simulink model "SAME70Q21B_MCPWM_MCLV2_PIM_DualShunt_R2018a"  (R2018a)
settings: Solver=FixedStepDiscrete  StartTime=0.0  StopTime=10.0  FixedStep=5e-5  RelTol=1e-3  EnableMultiTasking=on
undefined symbols (not defined in the file): A24, AD10, AD7, ADC0, DiscIntNeverNeededParam, gcbh, LQFP144, MCHP_AFEC_SAM7x_Callback, PA10, PA11, PA12, PA13, PA18, PA9, PB0, PB2, PB3, PD24, PD25, PD26, Pin, PWM0max0, SAME70Q21B, XData
libraries: MCHP_Blockset x10, simulink x9
(part 2 of 2)

== system SAME70Q21B_MCPWM_MCLV2_PIM_DualShunt_R2018a/Compute Voltage applied Within Alpha Beta Space1 ==
  Gain : Inport
  CosSin : Inport  Port=2
  DC Bus Voltage : Inport  Port=3
  Abs : Abs
  Delay : Delay  DelayLength=1  InitialCondition=0
  Product1 : Product  RndMeth=Zero  OutDataTypeStr=Inherit: Same as first input
  Product3 : Product  OutMin=[-24]  OutMax=[24]  RndMeth=Zero  OutDataTypeStr=Inherit: Same as first input
  ValphaBeta : Outport
  wires:
  Abs/1 -> Product1/2
  Gain/1 -> Abs/1
  CosSin/1 -> Delay/1
  Product3/1 -> ValphaBeta/1
  Product1/1 -> Product3/1
  DC Bus Voltage/1 -> Product3/2
  Delay/1 -> Product1/1

== system SAME70Q21B_MCPWM_MCLV2_PIM_DualShunt_R2018a/Invert Current Sign For reversed rotation1 ==
  Gain : Inport
  "Iab " : Inport  Port=2
  Compare To Zero1 : simulink/Logic and Bit Operations/Compare To Zero  relop=>=  OutDataTypeStr=boolean
  Gain4 : Gain  Gain=-1  RndMeth=Zero  SaturateOnIntegerOverflow=on  OutDataTypeStr=Inherit: Same as input
  Switch3 : Switch  Criteria=u2 ~= 0  Threshold=250
  "Iab_ " : Outport
  wires:
  "Iab "/1 -> Gain4/1, Switch3/1
  Gain/1 -> Compare To Zero1/1
  Switch3/1 -> "Iab_ "/1
  Compare To Zero1/1 -> Switch3/2
  Gain4/1 -> Switch3/3

== system SAME70Q21B_MCPWM_MCLV2_PIM_DualShunt_R2018a/OPEN Loop Startup sequence ==
  Constant1 : Constant  Value=149*2^-32  OutDataTypeStr=fixdt(0,32,32)  SampleTime=.00005
  Delay : Delay  DelayLength=1  InitialCondition=0
  Delay2 : Delay  DelayLength=1  InitialCondition=0
  Saturation : Saturate  UpperLimit=149*2^-32*3/.00005  LowerLimit=0
  Sum : Sum  Inputs=|++  AccumDataTypeStr=fixdt(0,32,32)  OutDataTypeStr=Inherit: Same as accumulator  RndMeth=Simplest
  Sum1 : Sum  Inputs=|++  AccumDataTypeStr=fixdt(0,32,32)  OutDataTypeStr=Inherit: Same as accumulator  RndMeth=Simplest
  Out1 : Outport
  wires:
  Delay/1 -> Sum/2
  Sum/1 -> Saturation/1  "Startup Ramp"
  Constant1/1 -> Sum/1
  Sum1/1 -> Out1/1, Delay2/1  "qAngle"
  Delay2/1 -> Sum1/2
  Saturation/1 -> Delay/1, Sum1/1

== system SAME70Q21B_MCPWM_MCLV2_PIM_DualShunt_R2018a/Scale ==
  In1 : Inport
  Data Type Conversion : DataTypeConversion  OutDataTypeStr=fixdt(1,32,31)
  Data Type Conversion1 : DataTypeConversion  OutDataTypeStr=fixdt(0,32,32)  ConvertRealWorld=Stored Integer (SI)
  Rate Transition2 : RateTransition
  Phase shift : Outport
  wires:
  In1/1 -> Data Type Conversion/1
  Data Type Conversion/1 -> Data Type Conversion1/1
  Data Type Conversion1/1 -> Rate Transition2/1
  Rate Transition2/1 -> Phase shift/1

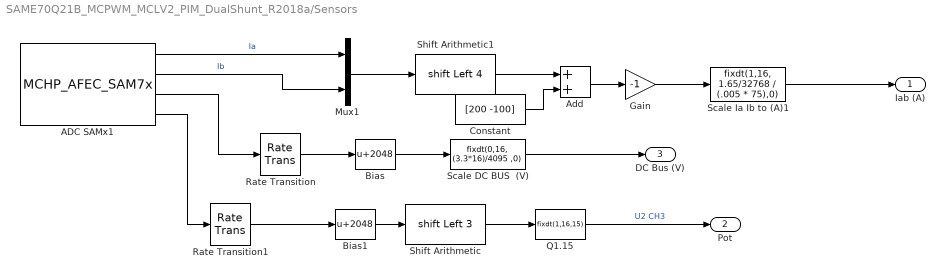
== system SAME70Q21B_MCPWM_MCLV2_PIM_DualShunt_R2018a/Sensors ==
  ADC SAMx1 : S-Function  Priority=-2000  AncestorBlock=MCHP_Blockset/Analog IO/ADC SAMx7  LoadFcn=|  InitFcn=MCHP_AFEC_SAM7x_Callback(gcbh,'InitFcn');  FunctionName=MCHP_AFEC_SAM7x  Parameters=MCHP_AFEC_SAM7x_Callback(gcbh,'S_INPUT'),MCHP_AFEC_SAM7x_Callback(gcbh,'S_OUTPUT'),MCHP_AFEC_SAM7x_Callback(gcbh,'S_INPUT_Size'),MCHP_AFEC_SAM7x_Callback(gcbh,'S_OUTPUT_Size'),MCHP_AFEC_SAM7x_Callback(gcbh,'S_ListCustomDatatype'),SampleTime,0  SFunctionDeploymentMode=off  EnableBusSupport=off  mask(ADC for SAMx7){AFECx=AFE Controller 0, SIGNMODE_SingleEnded=Signed    (int16), SIGNMODE_Differential=Unsigned (uint16), AFEC0_seq0=Dynamic Options, AFEC0_seq0_TXT=AD0 / PD30   &   AD6 / PA17, AFEC1_seq0=Dynamic Options, AFEC1_seq0_TXT=Not used, AFEC0_seq1=Dynamic Options, AFEC0_seq1_TXT=AD7 / PA18, AFEC1_seq1=Dynamic Options, AFEC1_seq1_TXT=Not used, AFEC0_seq2=Dynamic Options, AFEC0_seq2_TXT=AD10 / PB0, AFEC1_seq2=Dynamic Options, AFEC1_seq2_TXT=Not used, AFEC0_seq3=Dynamic Options, AFEC0_seq3_TXT=Not used, AFEC1_seq3=Dynamic Options, AFEC1_seq3_TXT=Not used, AFEC0_seq4=Dynamic Options, AFEC0_seq4_TXT=Not used, AFEC1_seq4=Dynamic Options, AFEC1_seq4_TXT=Not used, AFEC0_seq5=Dynamic Options, AFEC0_seq5_TXT=Not used, AFEC1_seq5=Dynamic Options, AFEC1_seq5_TXT=Not used, AFEC0_seq6=Dynamic Options, AFEC0_seq6_TXT=Not used, AFEC1_seq6=Dynamic Options, AFEC1_seq6_TXT=Not used, AFEC0_seq7=Dynamic Options, AFEC0_seq7_TXT=Not used, AFEC1_seq7=Dynamic Options, AFEC1_seq7_TXT=Not used, AFEC0_seq8=Dynamic Options, AFEC0_seq8_TXT=Not used, AFEC1_seq8=Dynamic Options, AFEC1_seq8_TXT=Not used, AFEC0_seq9=Dynamic Options, AFEC0_seq9_TXT=Not used, AFEC1_seq9=Dynamic Options, AFEC1_seq9_TXT=Not used, AFEC0_seq10=Dynamic Options, AFEC0_seq10_TXT=Not used, AFEC1_seq10=Dynamic Options, AFEC1_seq10_TXT=Not used, AFEC0_seq11=Dynamic Options, AFEC0_seq11_TXT=Not used, AFEC1_seq11=Dynamic Options, AFEC1_seq11_TXT=Not used, SampleTime=.00005, S_INPUT=[-1], S_INPUT_Size=[3], S_OUTPUT=[], S_OUTPUT_Size=[], S_ListCustomDatatype=S.S_ListCustomDatatype={};, evalin_ws=, MCHP_AFECC_CLOCK_REQUEST='', MCHP_AFECC_CLOCK_RESULT='', MCHP_USER_INTERRUPTS=0, MCHP_PORT={AD0 AFEC0}{AD0}15:2:P126;{AD6 AFEC0}{AD6}15:2:P17;{AD7 AFEC0}{AD7}15:2:P18;{AD10 AFEC0}{AD10}15:2:P32;, MCHP_MASTERLINK=SAME70Q21B_MCPWM_MCLV2_PIM_DualShunt_R2018a/Microchip Master, Rin=< 200 Ohm, RES=12-bit Standard, AFEC0_Synchronisation=Triggered by user defined source, AFEC0_Trig=PWM0 event line 0, AFEC0_TrigTimeStep=on, AFEC1_Synchronisation=Triggered by user defined source, AFEC1_Trig=PWM1 event line 0, AFEC1_TrigTimeStep=off, ADC_TrigInfo=0, AFEC0_seq0_GAIN=1, AFEC1_seq0_GAIN=1, AFEC0_seq1_GAIN=1, AFEC1_seq1_GAIN=1, AFEC0_seq2_GAIN=1, AFEC1_seq2_GAIN=1, AFEC0_seq3_GAIN=1, AFEC1_seq3_GAIN=1, AFEC0_seq4_GAIN=1, AFEC1_seq4_GAIN=1, AFEC0_seq5_GAIN=1, AFEC1_seq5_GAIN=1, AFEC0_seq6_GAIN=1, AFEC1_seq6_GAIN=1, AFEC0_seq7_GAIN=1, AFEC1_seq7_GAIN=1, AFEC0_seq8_GAIN=1, AFEC1_seq8_GAIN=1, AFEC0_seq9_GAIN=1, AFEC1_seq9_GAIN=1, AFEC0_seq10_GAIN=1, AFEC1_seq10_GAIN=1, AFEC0_seq11_GAIN=1, AFEC1_seq11_GAIN=1, AFEC0_seq0_OFFSET=0, AFEC1_seq0_OFFSET=0, AFEC0_seq1_OFFSET=0, AFEC1_seq1_OFFSET=0, AFEC0_seq2_OFFSET=0, AFEC1_seq2_OFFSET=0, AFEC0_seq3_OFFSET=0, AFEC1_seq3_OFFSET=0, AFEC0_seq4_OFFSET=0, AFEC1_seq4_OFFSET=0, AFEC0_seq5_OFFSET=0, AFEC1_seq5_OFFSET=0, AFEC0_seq6_OFFSET=0, AFEC1_seq6_OFFSET=0, AFEC0_seq7_OFFSET=0, AFEC1_seq7_OFFSET=0, AFEC0_seq8_OFFSET=0, AFEC1_seq8_OFFSET=0, AFEC0_seq9_OFFSET=0, AFEC1_seq9_OFFSET=0, AFEC0_seq10_OFFSET=0, AFEC1_seq10_OFFSET=0, AFEC0_seq11_OFFSET=0, AFEC1_seq11_OFFSET=0}
      | txt = get_param(gcbh,'evalin_ws');
      | evalin('base',txt);
      mask prompts: AFECx "Select ADC (AFEC) Controller :"; SIGNMODE_SingleEnded "Single-Ended conversion output are"; SIGNMODE_Differential "Differential conversions output are"; AFEC0_seq0 "AFEC0 seq 0"; AFEC0_seq0_TXT "sequence x"; AFEC1_seq0 "AFEC1 seq 0"; AFEC1_seq0_TXT "sequence x"; AFEC0_seq1 "AFEC0 seq 1"; AFEC0_seq1_TXT "sequence x"; AFEC1_seq1 "AFEC1 seq 1"; AFEC1_seq1_TXT "sequence x"; AFEC0_seq2 "AFEC0 seq 2"; AFEC0_seq2_TXT "sequence x"; AFEC1_seq2 "AFEC1 seq 2"; AFEC1_seq2_TXT "sequence x"; AFEC0_seq3 "AFEC0 seq 3"; AFEC0_seq3_TXT "sequence x"; AFEC1_seq3 "AFEC1 seq 3"; AFEC1_seq3_TXT "sequence x"; AFEC0_seq4 "AFEC0 seq 4"; AFEC0_seq4_TXT "sequence x"; AFEC1_seq4 "AFEC1 seq 4"; AFEC1_seq4_TXT "sequence x"; AFEC0_seq5 "AFEC0 seq 5"; AFEC0_seq5_TXT "sequence x"; AFEC1_seq5 "AFEC1 seq 5"; AFEC1_seq5_TXT "sequence x"; AFEC0_seq6 "AFEC0 seq 6"; AFEC0_seq6_TXT "sequence x"; AFEC1_seq6 "AFEC1 seq 6"; AFEC1_seq6_TXT "sequence x"; AFEC0_seq7 "AFEC0 seq 7"; AFEC0_seq7_TXT "sequence x"; AFEC1_seq7 "AFEC1 seq 7"; AFEC1_seq7_TXT "sequence x"; AFEC0_seq8 "AFEC0 seq 8"; AFEC0_seq8_TXT "sequence x"; AFEC1_seq8 "AFEC1 seq 8"; AFEC1_seq8_TXT "sequence x"; AFEC0_seq9 "AFEC0 seq 9"; AFEC0_seq9_TXT "sequence x"; AFEC1_seq9 "AFEC1 seq 9"; AFEC1_seq9_TXT "sequence x"; AFEC0_seq10 "AFEC0 seq 10"; AFEC0_seq10_TXT "sequence x"; AFEC1_seq10 "AFEC1 seq 10"; AFEC1_seq10_TXT "sequence x"; AFEC0_seq11 "AFEC0 seq 11"; AFEC0_seq11_TXT "sequence x"; AFEC1_seq11 "AFEC1 seq 11"; AFEC1_seq11_TXT "sequence x"; SampleTime "Block output sample time"; Rin "Input impedance (Tsamp=400(ns) ; Tconv=213.33(ns))"; RES "Resolution and Digital Filter"; AFEC0_Synchronisation "ADC Sample and Conversion"; AFEC0_Trig "User defined trigger (AFEC0):"; AFEC0_TrigTimeStep "The model base Time Step is triggered by the the last ADC conversion using this trigger"; AFEC1_Synchronisation "ADC Sample and Conversion"; AFEC1_Trig "User defined trigger (AFEC1):"; AFEC1_TrigTimeStep "The model base Time Step is triggered by the the last ADC conversion using this trigger"; ADC_TrigInfo "ADC Trigger Info"; AFEC0_seq0_GAIN "AD0 - PD30 Gain"; AFEC1_seq0_GAIN "AD0 - PB1 Gain"; AFEC0_seq1_GAIN "AD1 - PA21 Gain"; AFEC1_seq1_GAIN "AD1 - PC13 Gain"; AFEC0_seq2_GAIN "AD2 - PB3 Gain"; AFEC1_seq2_GAIN "AD2 - PC15 Gain"; AFEC0_seq3_GAIN "AD3 - PE5 Gain"; AFEC1_seq3_GAIN "AD3 - PC12 Gain"; AFEC0_seq4_GAIN "AD4 - PE4 Gain"; AFEC1_seq4_GAIN "AD4 - PC29 Gain"; AFEC0_seq5_GAIN "AD5 - PB2 Gain"; AFEC1_seq5_GAIN "AD5 - PC30 Gain"; AFEC0_seq6_GAIN "AD6 - PA17 Gain"; AFEC1_seq6_GAIN "AD6 - PC31 Gain"; AFEC0_seq7_GAIN "AD7 - PA18 Gain"; AFEC1_seq7_GAIN "AD7 - PC26 Gain"; AFEC0_seq8_GAIN "AD8 - PA19 Gain"; AFEC1_seq8_GAIN "AD8 - PC27 Gain"; AFEC0_seq9_GAIN "AD9 - PA20 Gain"; AFEC1_seq9_GAIN "AD9 - PC0 Gain"; AFEC0_seq10_GAIN "AD10 - PB0 Gain"; AFEC1_seq10_GAIN "AD10 - PE3 Gain"; AFEC0_seq11_GAIN "AD11 - T Gain"; AFEC1_seq11_GAIN "AD11 - PE0 Gain"; AFEC0_seq0_OFFSET "AD0 - PD30 Offset within [-512 511]"; AFEC1_seq0_OFFSET "AD0 - PB1 Offset within [-512 511]"; AFEC0_seq1_OFFSET "AD1 - PA21 Offset within [-512 511]"; AFEC1_seq1_OFFSET "AD1 - PC13 Offset within [-512 511]"; AFEC0_seq2_OFFSET "AD2 - PB3 Offset within [-512 511]"; AFEC1_seq2_OFFSET "AD2 - PC15 Offset within [-512 511]"; AFEC0_seq3_OFFSET "AD3 - PE5 Offset within [-512 511]"; AFEC1_seq3_OFFSET "AD3 - PC12 Offset within [-512 511]"; AFEC0_seq4_OFFSET "AD4 - PE4 Offset within [-512 511]"; AFEC1_seq4_OFFSET "AD4 - PC29 Offset within [-512 511]"; AFEC0_seq5_OFFSET "AD5 - PB2 Offset within [-512 511]"; AFEC1_seq5_OFFSET "AD5 - PC30 Offset within [-512 511]"; AFEC0_seq6_OFFSET "AD6 - PA17 Offset within [-512 511]"; AFEC1_seq6_OFFSET "AD6 - PC31 Offset within [-512 511]"; AFEC0_seq7_OFFSET "AD7 - PA18 Offset within [-512 511]"; AFEC1_seq7_OFFSET "AD7 - PC26 Offset within [-512 511]"; AFEC0_seq8_OFFSET "AD8 - PA19 Offset within [-512 511]"; AFEC1_seq8_OFFSET "AD8 - PC27 Offset within [-512 511]"; AFEC0_seq9_OFFSET "AD9 - PA20 Offset within [-512 511]"; AFEC1_seq9_OFFSET "AD9 - PC0 Offset within [-512 511]"; AFEC0_seq10_OFFSET "AD10 - PB0 Offset within [-512 511]"; AFEC1_seq10_OFFSET "AD10 - PE3 Offset within [-512 511]"; AFEC0_seq11_OFFSET "AD11 - T Offset within [-512 511]"; AFEC1_seq11_OFFSET "AD11 - PE0 Offset within [-512 511]"
      mask help:
      | Configure the Analog Front End Controller (AFEC).
      |
      | Two AFEC modules can be configured independantly using two ADC blocks.
      | They will have common parameters when set with one common block.
      |
      | The 11 analog input pins are different for each AFEC.
      |
      | The sequence set in the block is listed in sampling chronological order.
      mask init:
      | MCHP_AFEC_SAM7x_Callback(gcbh,'INITIALISATION');
      settings: CopyFcn=MCHP_AFEC_SAM7x_Callback(gcbh,'CopyFcn');  PreSaveFcn=MCHP_Fun.PreSaveFcn_DynamicOptions(gcbh);  OpenFcn=MCHP_AFEC_SAM7x_Callback(gcbh,'OPEN');
      mask TypeOptions AFECx: AFE Controller 0 | AFE Controller 1 | AFE Controller 0 & 1
      mask Callback AFECx: MCHP_AFEC_SAM7x_Callback(gcbh,'UpdateGUI');
      mask TypeOptions SIGNMODE_SingleEnded: Unsigned (uint16) | Signed    (int16)
      mask TypeOptions SIGNMODE_Differential: Unsigned (uint16) | Signed    (int16)
      mask TypeOptions AFEC0_seq0: Dynamic Options
      mask Callback AFEC0_seq0: MCHP_AFEC_SAM7x_Callback(gcbh,'UpdateGUI');
      mask Callback AFEC0_seq0_TXT: MCHP_AFEC_SAM7x_Callback(gcbh,'UpdateGUI');
      mask TypeOptions AFEC1_seq0: Dynamic Options
      mask Callback AFEC1_seq0: MCHP_AFEC_SAM7x_Callback(gcbh,'UpdateGUI');
      mask Callback AFEC1_seq0_TXT: MCHP_AFEC_SAM7x_Callback(gcbh,'UpdateGUI');
      mask TypeOptions AFEC0_seq1: Dynamic Options
      mask Callback AFEC0_seq1: MCHP_AFEC_SAM7x_Callback(gcbh,'UpdateGUI');
      mask Callback AFEC0_seq1_TXT: MCHP_AFEC_SAM7x_Callback(gcbh,'UpdateGUI');
      mask TypeOptions AFEC1_seq1: Dynamic Options
      mask Callback AFEC1_seq1: MCHP_AFEC_SAM7x_Callback(gcbh,'UpdateGUI');
      mask Callback AFEC1_seq1_TXT: MCHP_AFEC_SAM7x_Callback(gcbh,'UpdateGUI');
      mask TypeOptions AFEC0_seq2: Dynamic Options
      mask Callback AFEC0_seq2_TXT: MCHP_AFEC_SAM7x_Callback(gcbh,'UpdateGUI');
      mask TypeOptions AFEC1_seq2: Dynamic Options
      mask Callback AFEC1_seq2_TXT: MCHP_AFEC_SAM7x_Callback(gcbh,'UpdateGUI');
      mask TypeOptions AFEC0_seq3: Dynamic Options
      mask Callback AFEC0_seq3: MCHP_AFEC_SAM7x_Callback(gcbh,'UpdateGUI');
      mask Callback AFEC0_seq3_TXT: MCHP_AFEC_SAM7x_Callback(gcbh,'UpdateGUI');
      mask TypeOptions AFEC1_seq3: Dynamic Options
      mask Callback AFEC1_seq3: MCHP_AFEC_SAM7x_Callback(gcbh,'UpdateGUI');
      mask Callback AFEC1_seq3_TXT: MCHP_AFEC_SAM7x_Callback(gcbh,'UpdateGUI');
      mask TypeOptions AFEC0_seq4: Dynamic Options
      mask Callback AFEC0_seq4: MCHP_AFEC_SAM7x_Callback(gcbh,'UpdateGUI');
      mask Callback AFEC0_seq4_TXT: MCHP_AFEC_SAM7x_Callback(gcbh,'UpdateGUI');
      mask TypeOptions AFEC1_seq4: Dynamic Options
      mask Callback AFEC1_seq4: MCHP_AFEC_SAM7x_Callback(gcbh,'UpdateGUI');
      mask Callback AFEC1_seq4_TXT: MCHP_AFEC_SAM7x_Callback(gcbh,'UpdateGUI');
      mask TypeOptions AFEC0_seq5: Dynamic Options
      mask Callback AFEC0_seq5: MCHP_AFEC_SAM7x_Callback(gcbh,'UpdateGUI');
      mask Callback AFEC0_seq5_TXT: MCHP_AFEC_SAM7x_Callback(gcbh,'UpdateGUI');
      mask TypeOptions AFEC1_seq5: Dynamic Options
      mask Callback AFEC1_seq5: MCHP_AFEC_SAM7x_Callback(gcbh,'UpdateGUI');
      mask Callback AFEC1_seq5_TXT: MCHP_AFEC_SAM7x_Callback(gcbh,'UpdateGUI');
      mask TypeOptions AFEC0_seq6: Dynamic Options
      mask Callback AFEC0_seq6: MCHP_AFEC_SAM7x_Callback(gcbh,'UpdateGUI');
      mask Callback AFEC0_seq6_TXT: MCHP_AFEC_SAM7x_Callback(gcbh,'UpdateGUI');
      mask TypeOptions AFEC1_seq6: Dynamic Options
      mask Callback AFEC1_seq6: MCHP_AFEC_SAM7x_Callback(gcbh,'UpdateGUI');
      mask Callback AFEC1_seq6_TXT: MCHP_AFEC_SAM7x_Callback(gcbh,'UpdateGUI');
      mask TypeOptions AFEC0_seq7: Dynamic Options
      mask Callback AFEC0_seq7: MCHP_AFEC_SAM7x_Callback(gcbh,'UpdateGUI');
      mask Callback AFEC0_seq7_TXT: MCHP_AFEC_SAM7x_Callback(gcbh,'UpdateGUI');
      mask TypeOptions AFEC1_seq7: Dynamic Options
      mask Callback AFEC1_seq7: MCHP_AFEC_SAM7x_Callback(gcbh,'UpdateGUI');
      mask Callback AFEC1_seq7_TXT: MCHP_AFEC_SAM7x_Callback(gcbh,'UpdateGUI');
      mask TypeOptions AFEC0_seq8: Dynamic Options
      mask Callback AFEC0_seq8: MCHP_AFEC_SAM7x_Callback(gcbh,'UpdateGUI');
      mask Callback AFEC0_seq8_TXT: MCHP_AFEC_SAM7x_Callback(gcbh,'UpdateGUI');
      mask TypeOptions AFEC1_seq8: Dynamic Options
      mask Callback AFEC1_seq8: MCHP_AFEC_SAM7x_Callback(gcbh,'UpdateGUI');
      mask Callback AFEC1_seq8_TXT: MCHP_AFEC_SAM7x_Callback(gcbh,'UpdateGUI');
      mask TypeOptions AFEC0_seq9: Dynamic Options
      mask Callback AFEC0_seq9: MCHP_AFEC_SAM7x_Callback(gcbh,'UpdateGUI');
      mask Callback AFEC0_seq9_TXT: MCHP_AFEC_SAM7x_Callback(gcbh,'UpdateGUI');
      mask TypeOptions AFEC1_seq9: Dynamic Options
      mask Callback AFEC1_seq9: MCHP_AFEC_SAM7x_Callback(gcbh,'UpdateGUI');
      mask Callback AFEC1_seq9_TXT: MCHP_AFEC_SAM7x_Callback(gcbh,'UpdateGUI');
      mask TypeOptions AFEC0_seq10: Dynamic Options
      mask Callback AFEC0_seq10: MCHP_AFEC_SAM7x_Callback(gcbh,'UpdateGUI');
      mask Callback AFEC0_seq10_TXT: MCHP_AFEC_SAM7x_Callback(gcbh,'UpdateGUI');
      mask TypeOptions AFEC1_seq10: Dynamic Options
      mask Callback AFEC1_seq10: MCHP_AFEC_SAM7x_Callback(gcbh,'UpdateGUI');
      mask Callback AFEC1_seq10_TXT: MCHP_AFEC_SAM7x_Callback(gcbh,'UpdateGUI');
      mask TypeOptions AFEC0_seq11: Dynamic Options
      mask Callback AFEC0_seq11: MCHP_AFEC_SAM7x_Callback(gcbh,'UpdateGUI');
      mask Callback AFEC0_seq11_TXT: MCHP_AFEC_SAM7x_Callback(gcbh,'UpdateGUI');
      mask TypeOptions AFEC1_seq11: Dynamic Options
      mask Callback AFEC1_seq11: MCHP_AFEC_SAM7x_Callback(gcbh,'UpdateGUI');
      mask Callback AFEC1_seq11_TXT: MCHP_AFEC_SAM7x_Callback(gcbh,'UpdateGUI');
      mask TypeOptions Rin: < 200 Ohm | < 500 Ohm | < 1    kOhm | < 2    kOhm | < 5    kOhm | < 10   kOhm | < 20   kOhm | < 50   kOhm | < 100  kOhm | < 200  kOhm | < 500  kOhm | max sampling time
      mask TypeOptions RES: 10-bit Low Resolution | 12-bit Standard | 13-bit (Average 4 conversions) | 14-bit (Average 16 conversions) | 15-bit (Average 64 conversions) | 16-bit (Average 256 conversions)
      mask TypeOptions AFEC0_Synchronisation: Software triggered after reading last converted value | Triggered by user defined source | Free Run. Output is last converted value
      mask Callback AFEC0_Synchronisation: MCHP_AFEC_SAM7x_Callback(gcbh,'UpdateGUI');
      mask TypeOptions AFEC0_Trig: AFE0_ADTRG input pin | PWM0 event line 0 | PWM0 event line 1 | Timer Counter Channel 0 | Timer Counter Channel 1 | Timer Counter Channel 2 | Analog Comparator
      mask TypeOptions AFEC1_Synchronisation: Software triggered after reading last converted value | Triggered by user defined source | Free Run. Output is last converted value
      mask Callback AFEC1_Synchronisation: MCHP_AFEC_SAM7x_Callback(gcbh,'UpdateGUI');
      mask TypeOptions AFEC1_Trig: AFE1_ADTRG input pin | PWM1 event line 0 | PWM1 event line 1 | Timer Counter Channel 3 | Timer Counter Channel 4 | Timer Counter Channel 5 | Analog Comparator
      mask TypeOptions AFEC0_seq0_GAIN: 1 | 2 | 4
      mask TypeOptions AFEC1_seq0_GAIN: 1 | 2 | 4
      mask TypeOptions AFEC0_seq1_GAIN: 1 | 2 | 4
      mask TypeOptions AFEC1_seq1_GAIN: 1 | 2 | 4
      mask TypeOptions AFEC0_seq2_GAIN: 1 | 2 | 4
      mask TypeOptions AFEC1_seq2_GAIN: 1 | 2 | 4
      mask TypeOptions AFEC0_seq3_GAIN: 1 | 2 | 4
      mask TypeOptions AFEC1_seq3_GAIN: 1 | 2 | 4
      mask TypeOptions AFEC0_seq4_GAIN: 1 | 2 | 4
      mask TypeOptions AFEC1_seq4_GAIN: 1 | 2 | 4
      mask TypeOptions AFEC0_seq5_GAIN: 1 | 2 | 4
      mask TypeOptions AFEC1_seq5_GAIN: 1 | 2 | 4
      mask TypeOptions AFEC0_seq6_GAIN: 1 | 2 | 4
      mask TypeOptions AFEC1_seq6_GAIN: 1 | 2 | 4
      mask TypeOptions AFEC0_seq7_GAIN: 1 | 2 | 4
      mask TypeOptions AFEC1_seq7_GAIN: 1 | 2 | 4
      mask TypeOptions AFEC0_seq8_GAIN: 1 | 2 | 4
      mask TypeOptions AFEC1_seq8_GAIN: 1 | 2 | 4
      mask TypeOptions AFEC0_seq9_GAIN: 1 | 2 | 4
      mask TypeOptions AFEC1_seq9_GAIN: 1 | 2 | 4
      mask TypeOptions AFEC0_seq10_GAIN: 1 | 2 | 4
      mask TypeOptions AFEC1_seq10_GAIN: 1 | 2 | 4
      mask TypeOptions AFEC0_seq11_GAIN: 1 | 2 | 4
      mask TypeOptions AFEC1_seq11_GAIN: 1 | 2 | 4
      mask DialogControl ParameterTabVar0 Prompt: Analog Channels
      mask DialogControl ParameterTabVar01 Prompt: Options
      mask DialogControl ParameterTabVar012 Prompt: Gain
      mask DialogControl ParameterTabVar0123 Prompt: Offset
      mask Display:
      | fprintf(['AFEC SAMx7\n' AFECx(4:end)]);
      | port_label('output',1,'PD30');
      | port_label('output',2,'PA17');
      | port_label('output',3,'PA18');
      | port_label('output',4,'PB0');
  Add : Sum  SaturateOnIntegerOverflow=on  OutDataTypeStr=Inherit: Same as first input
  Bias : Bias  Bias=2048
  Bias1 : Bias  Bias=2048
  Constant : Constant  Value=[200 -100]  OutDataTypeStr=int16
  Gain : Gain  Gain=-1  SaturateOnIntegerOverflow=on  OutDataTypeStr=Inherit: Same as input
  Mux1 : Mux  Inputs=2
  Q1.15 : DataTypeConversion  OutDataTypeStr=fixdt(1,16,15)  ConvertRealWorld=Stored Integer (SI)
  Rate Transition : RateTransition  OutPortSampleTime=.001
  Rate Transition1 : RateTransition  OutPortSampleTime=.001
  Scale DC BUS  (V) : DataTypeConversion  OutDataTypeStr=fixdt(0,16, (3.3*16)/4095 ,0)  ConvertRealWorld=Stored Integer (SI)
  Scale Ia Ib to (A)1 : DataTypeConversion  OutDataTypeStr=fixdt(1,16, 1.65/32768 / (.005 * 75),0)  ConvertRealWorld=Stored Integer (SI)
  Shift Arithmetic : ArithShift  BitShiftNumber=3  BitShiftDirection=Left
  Shift Arithmetic1 : ArithShift  BitShiftNumber=4  BitShiftDirection=Left
  Iab (A) : Outport
  Pot : Outport  Port=2
  DC Bus (V) : Outport  Port=3
  wires:
  Q1.15/1 -> Pot/1  "U2 CH3"
  Mux1/1 -> Shift Arithmetic1/1
  Scale Ia Ib to (A)1/1 -> Iab (A)/1
  Scale DC BUS  (V)/1 -> DC Bus (V)/1
  ADC SAMx1/4 -> Rate Transition1/1
  Shift Arithmetic/1 -> Q1.15/1
  Bias/1 -> Scale DC BUS  (V)/1
  ADC SAMx1/3 -> Rate Transition/1
  Bias1/1 -> Shift Arithmetic/1
  Rate Transition/1 -> Bias/1
  Rate Transition1/1 -> Bias1/1
  ADC SAMx1/2 -> Mux1/2  "Ib"
  Shift Arithmetic1/1 -> Add/1
  Add/1 -> Gain/1
  ADC SAMx1/1 -> Mux1/1  "Ia"
  Constant/1 -> Add/2
  Gain/1 -> Scale Ia Ib to (A)1/1

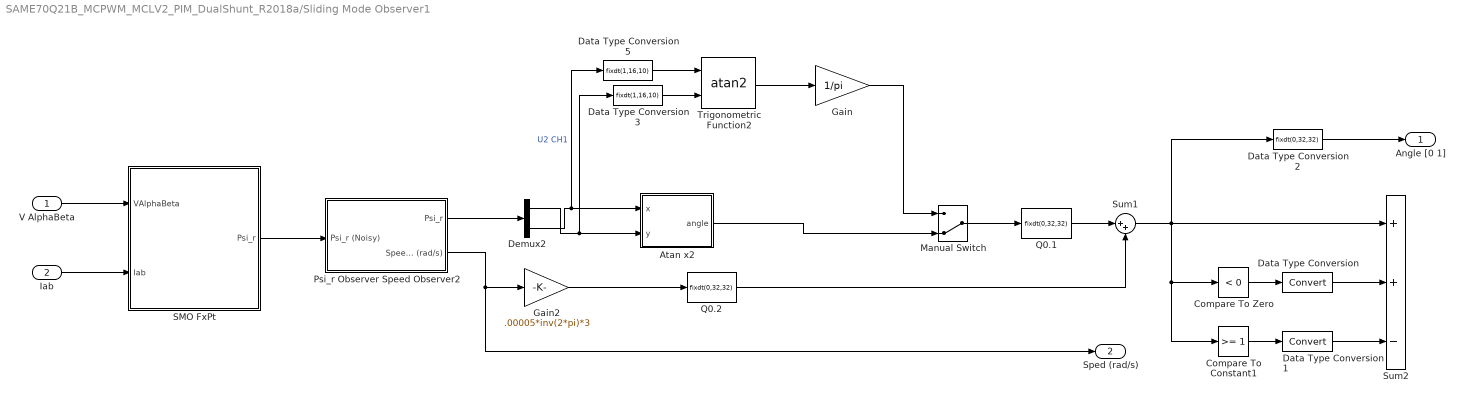
== system SAME70Q21B_MCPWM_MCLV2_PIM_DualShunt_R2018a/Sliding Mode Observer1 ==
  V AlphaBeta : Inport
  Iab : Inport  Port=2
  Atan x2 : Subsystem  AncestorBlock=Lib_MCHP_BLKDEMO_Motor/Atan x2
  Compare To Constant1 : simulink/Logic and Bit Operations/Compare To Constant  relop=>=  const=1  OutDataTypeStr=boolean
  Compare To Zero : simulink/Logic and Bit Operations/Compare To Zero  relop=<  OutDataTypeStr=boolean
  Data Type Conversion : DataTypeConversion  RndMeth=Zero
  Data Type Conversion1 : DataTypeConversion  RndMeth=Zero
  Data Type Conversion2 : DataTypeConversion  OutDataTypeStr=fixdt(0,32,32)  RndMeth=Zero
  Data Type Conversion3 : DataTypeConversion  OutDataTypeStr=fixdt(1,16,10)  RndMeth=Zero
  Data Type Conversion5 : DataTypeConversion  OutDataTypeStr=fixdt(1,16,10)  RndMeth=Zero
  Demux2 : Demux  Outputs=2
  Gain : Gain  Gain=1/pi  OutDataTypeStr=fixdt(1,32,31)  RndMeth=Zero
  Gain2 : Gain  Gain=.00005*inv(2*pi)*3  OutDataTypeStr=fixdt(1,32,31)  RndMeth=Zero
  Manual Switch : ManualSwitch  CurrentSetting=0
  Psi_r Observer Speed Observer2 : Subsystem
  Q0.1 : DataTypeConversion  OutDataTypeStr=fixdt(0,32,32)  ConvertRealWorld=Stored Integer (SI)  RndMeth=Simplest
  Q0.2 : DataTypeConversion  OutDataTypeStr=fixdt(0,32,32)  ConvertRealWorld=Stored Integer (SI)  RndMeth=Simplest
  SMO FxPt : Subsystem
  Sum1 : Sum  Inputs=|++  OutDataTypeStr=Inherit: Same as accumulator  RndMeth=Zero
  Sum2 : Sum  Inputs=++-  OutDataTypeStr=Inherit: Same as accumulator  RndMeth=Zero
  Trigonometric Function2 : Trigonometry  Operator=atan2  ApproximationMethod=CORDIC  NumberOfIterations=10  OutputSignalType=real
  Angle [0 1] : Outport
  Sped (rad/s) : Outport  Port=2
  wires:
  Data Type Conversion2/1 -> Angle [0 1]/1
  Trigonometric Function2/1 -> Gain/1
  Data Type Conversion1/1 -> Sum2/3
  Data Type Conversion/1 -> Sum2/2
  Compare To Constant1/1 -> Data Type Conversion1/1
  Compare To Zero/1 -> Data Type Conversion/1
  Gain/1 -> Manual Switch/1
  Atan x2/1(angle) -> Manual Switch/2
  Demux2/2 -> Data Type Conversion5/1, Atan x2/1(x)  "U2 CH1"
  Manual Switch/1 -> Q0.1/1
  Sum1/1 -> Compare To Zero/1, Compare To Constant1/1, Data Type Conversion2/1, Sum2/1
  Iab/1 -> SMO FxPt/2(Iab)
  Psi_r Observer Speed Observer2/2(Speed we (rad/s)) -> Gain2/1, Sped (rad/s)/1
  SMO FxPt/1(Psi_r) -> Psi_r Observer Speed Observer2/1(Psi_r (Noisy))
  V AlphaBeta/1 -> SMO FxPt/1(VAlphaBeta)
  Psi_r Observer Speed Observer2/1(Psi_r) -> Demux2/1
  Demux2/1 -> Atan x2/2(y), Data Type Conversion3/1
  Gain2/1 -> Q0.2/1
  Q0.1/1 -> Sum1/1
  Data Type Conversion5/1 -> Trigonometric Function2/1
  Data Type Conversion3/1 -> Trigonometric Function2/2
  Q0.2/1 -> Sum1/2

== system SAME70Q21B_MCPWM_MCLV2_PIM_DualShunt_R2018a/Subsystem1 ==
  OL : Inport
  CL : Inport  Port=2
  Rate Transition10 : RateTransition
  Switch Startup ramp Angle then Estimated Angle or QEI : Switch  Criteria=u2 ~= 0  Threshold=250
  OL/CL : Outport
  wires:
  [CL] -> Rate Transition10/1
  Rate Transition10/1 -> Switch Startup ramp Angle then Estimated Angle or QEI/2
  Switch Startup ramp Angle then Estimated Angle or QEI/1 -> OL/CL/1
  OL/1 -> Switch Startup ramp Angle then Estimated Angle or QEI/3
  CL/1 -> Switch Startup ramp Angle then Estimated Angle or QEI/1

== system SAME70Q21B_MCPWM_MCLV2_PIM_DualShunt_R2018a/Subsystem2 ==
  CL : Inport
  OL : Inport  Port=2
  Rate Transition10 : RateTransition
  Switch Startup ramp Angle then Estimated Angle or QEI : Switch  Criteria=u2 ~= 0  Threshold=250
  OL/CL : Outport
  wires:
  CL/1 -> Switch Startup ramp Angle then Estimated Angle or QEI/1
  OL/1 -> Switch Startup ramp Angle then Estimated Angle or QEI/3
  Rate Transition10/1 -> Switch Startup ramp Angle then Estimated Angle or QEI/2
  [CL] -> Rate Transition10/1
  Switch Startup ramp Angle then Estimated Angle or QEI/1 -> OL/CL/1

== system SAME70Q21B_MCPWM_MCLV2_PIM_DualShunt_R2018a/Switch from OpenLoop to Closed Loop ==
  Speed : Inport
  Abs : Abs
  Delay1 : Delay  DelayLength=1  InitialCondition=[0]
  Logical Operator1 : Logic  Operator=OR  AllPortsSameDT=off  OutDataTypeStr=boolean
  Rate Transition8 : RateTransition  OutPortSampleTime=.01
  Switching Speed (rad/s Electrical) : simulink/Logic and Bit Operations/Compare To Constant  relop=>  const=100  OutDataTypeStr=boolean
  ClosedLoop 0/1 : Outport
  wires:
  Abs/1 -> Switching Speed (rad/s Electrical)/1
  Speed/1 -> Rate Transition8/1
  Rate Transition8/1 -> Abs/1
  Delay1/1 -> Logical Operator1/1, ClosedLoop 0/1/1
  Switching Speed (rad/s Electrical)/1 -> Logical Operator1/2
  Logical Operator1/1 -> Delay1/1

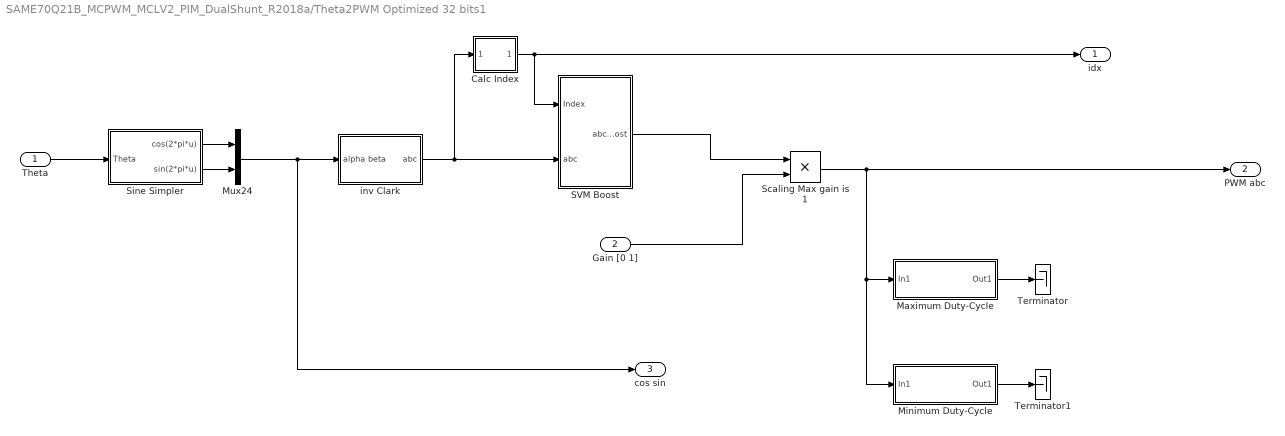
== system SAME70Q21B_MCPWM_MCLV2_PIM_DualShunt_R2018a/Theta2PWM Optimized 32 bits1 ==
  Theta : Inport
  Gain [0 1] : Inport  Port=2  OutMax=[PWM0max0/2]
  Calc Index : Subsystem
  Maximum Duty-Cycle : Subsystem
  Minimum Duty-Cycle : Subsystem
  Mux24 : Mux  Inputs=2
  SVM Boost : Subsystem
  Scaling Max gain is 1 : Product  Inputs=**  OutDataTypeStr=double
  Sine Simpler : Subsystem
  Terminator : Terminator
  Terminator1 : Terminator
  inv Clark : Subsystem
  idx : Outport
  PWM abc : Outport  Port=2
  cos sin : Outport  Port=3
  wires:
  Mux24/1 -> inv Clark/1(alpha beta), cos sin/1
  SVM Boost/1(abc boost) -> Scaling Max gain is 1/1
  Sine Simpler/2(sin(2*pi*u)) -> Mux24/2
  Sine Simpler/1(cos(2*pi*u)) -> Mux24/1
  Theta/1 -> Sine Simpler/1(Theta)
  inv Clark/1(abc) -> SVM Boost/2(abc), Calc Index/1(In1)
  Calc Index/1(Idx) -> idx/1, SVM Boost/1(Index)
  Gain [0 1]/1 -> Scaling Max gain is 1/2
  Maximum Duty-Cycle/1(Out1) -> Terminator/1
  Minimum Duty-Cycle/1(Out1) -> Terminator1/1
  Scaling Max gain is 1/1 -> PWM abc/1, Maximum Duty-Cycle/1(In1), Minimum Duty-Cycle/1(In1)

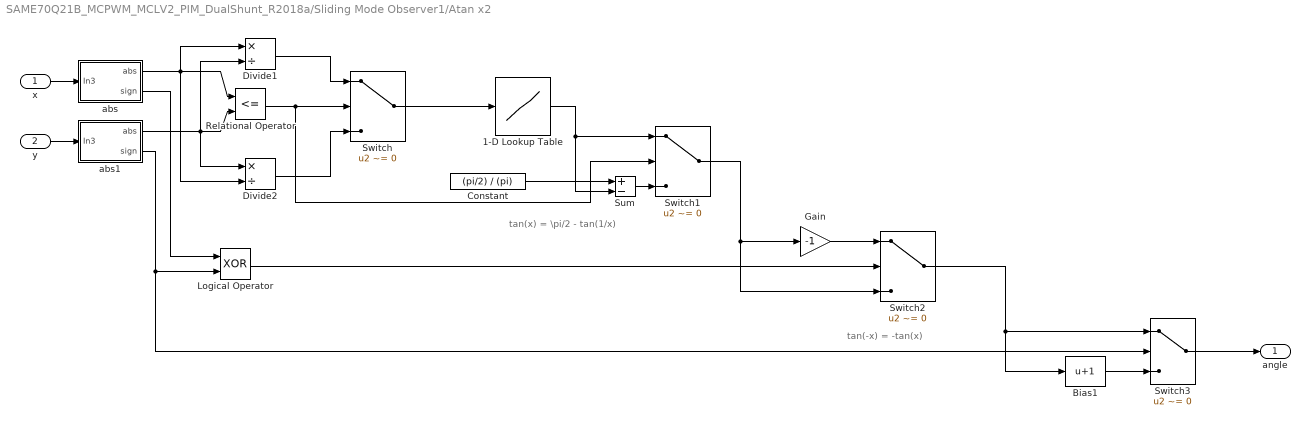
== system SAME70Q21B_MCPWM_MCLV2_PIM_DualShunt_R2018a/Sliding Mode Observer1/Atan x2 ==
  note: tan(x) = \pi/2 - tan(1/x)
  note: tan(-x) = -tan(x)
  x : Inport
  y : Inport  Port=2
  1-D Lookup Table : Lookup_n-D  NumberOfTableDimensions=1  BreakpointsSpecification=Even spacing  BreakpointsForDimension1=[0:2^-8:1]  BreakpointsForDimension1FirstPoint=0  BreakpointsForDimension1Spacing=2^-8  IndexSearchMethod=Evenly spaced points  BeginIndexSearchUsingPreviousIndexResult=on  Table=atan([0:2^-8:1])/(pi)  TableDataTypeStr=fixdt(1,32,31)  InterpMethod=Flat  ExtrapMethod=Clip  RemoveProtectionInput=on  UseLastTableValue=on  OutDataTypeStr=fixdt(1,32,31)  RndMeth=Simplest  InputSameDT=on  LockScale=on
  Bias1 : Bias  Bias=1
  Constant : Constant  Value=(pi/2) / (pi)  OutDataTypeStr=Inherit: Inherit via back propagation
  Divide1 : Product  Inputs=*/  OutDataTypeStr=fixdt(0,16,15)
  Divide2 : Product  Inputs=*/  OutDataTypeStr=fixdt(0,16,15)
  Gain : Gain  Gain=-1  OutDataTypeStr=Inherit: Same as input
  Logical Operator : Logic  Operator=XOR  AllPortsSameDT=off  OutDataTypeStr=boolean
  Relational Operator : RelationalOperator  Operator=<=  OutDataTypeStr=boolean  RndMeth=Nearest
  Sum : Sum  Inputs=+-
  Switch{,1..3} (4 alike) : Switch  Criteria=u2 ~= 0
  abs : Subsystem
  abs1 : Subsystem
  angle : Outport
  wires:
  Gain/1 -> Switch2/1
  Bias1/1 -> Switch3/3
  Switch3/1 -> angle/1
  Switch2/1 -> Switch3/1, Bias1/1
  Relational Operator/1 -> Switch/2, Switch1/2
  Divide2/1 -> Switch/3
  Divide1/1 -> Switch/1
  Switch/1 -> 1-D Lookup Table/1
  1-D Lookup Table/1 -> Switch1/1, Sum/2
  Constant/1 -> Sum/1
  Sum/1 -> Switch1/3
  abs/1(abs) -> Relational Operator/1, Divide1/1, Divide2/2
  x/1 -> abs/1(In3)
  abs1/1(abs) -> Relational Operator/2, Divide2/1, Divide1/2
  y/1 -> abs1/1(In3)
  abs/2(sign) -> Logical Operator/1
  abs1/2(sign) -> Logical Operator/2, Switch3/2
  Logical Operator/1 -> Switch2/2
  Switch1/1 -> Gain/1, Switch2/3

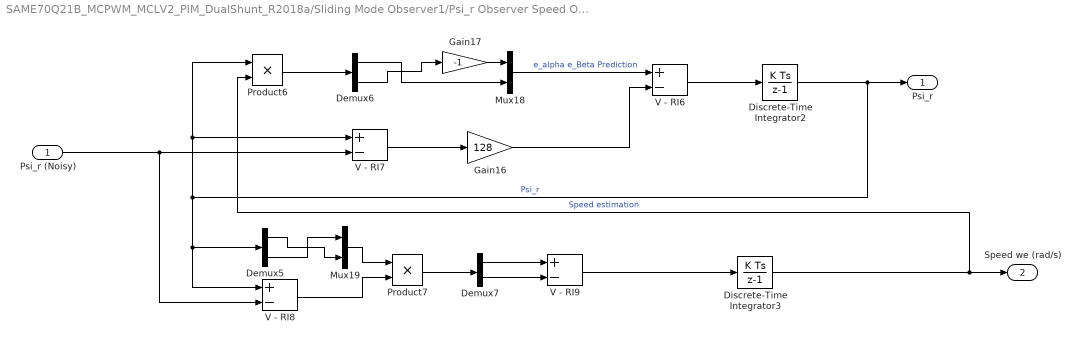
== system SAME70Q21B_MCPWM_MCLV2_PIM_DualShunt_R2018a/Sliding Mode Observer1/Psi_r Observer Speed Observer2 ==
  Psi_r (Noisy) : Inport
  Demux5 : Demux  Outputs=2
  Demux6 : Demux  Outputs=2
  Demux7 : Demux  Outputs=2
  Discrete-Time Integrator2 : DiscreteIntegrator  gainval=1  SampleTime=-1  OutMin=-24  OutMax=24  RndMeth=Zero  UpperSaturationLimit=15  LowerSaturationLimit=-15  ICPrevOutput=DiscIntNeverNeededParam  ICPrevScaledInput=DiscIntNeverNeededParam
  Discrete-Time Integrator3 : DiscreteIntegrator  gainval=1000  SampleTime=-1  OutMin=-5300 * 5 * (2*pi) / 60  OutMax=5300 * 5 * (2*pi) / 60  RndMeth=Zero  StateName=Speed  ICPrevOutput=DiscIntNeverNeededParam  ICPrevScaledInput=DiscIntNeverNeededParam
  Gain16 : Gain  Gain=128  OutMin=[-24*2*128]  OutMax=[24*2*128]  RndMeth=Zero
  Gain17 : Gain  Gain=-1  OutDataTypeStr=Inherit: Same as input
  Mux18 : Mux  Inputs=2
  Mux19 : Mux  Inputs=2
  Product6 : Product  RndMeth=Zero
  Product7 : Product  OutMin=[-24*24]  OutMax=24*24  RndMeth=Zero
  V - RI6 : Sum  Inputs=+-  OutDataTypeStr=Inherit: Same as accumulator  RndMeth=Zero
  V - RI7 : Sum  Inputs=+-  OutMin=[-24*2]  OutMax=[24*2]  RndMeth=Zero
  V - RI8 : Sum  Inputs=+-  OutDataTypeStr=Inherit: Same as accumulator  RndMeth=Zero
  V - RI9 : Sum  Inputs=+-  OutMin=[-24*24*2]  OutMax=[-24*24*2]  RndMeth=Zero  InputSameDT=on
  Psi_r : Outport
  Speed we (rad/s) : Outport  Port=2
  wires:
  V - RI9/1 -> Discrete-Time Integrator3/1
  V - RI6/1 -> Discrete-Time Integrator2/1
  V - RI7/1 -> Gain16/1
  Mux18/1 -> V - RI6/1  "e_alpha e_Beta Prediction"
  Demux5/2 -> Mux19/1
  Mux19/1 -> Product7/1
  V - RI8/1 -> Product7/2
  Product7/1 -> Demux7/1
  Demux7/1 -> V - RI9/1
  Demux7/2 -> V - RI9/2
  Product6/1 -> Demux6/1
  Gain17/1 -> Mux18/1
  Discrete-Time Integrator3/1 -> Product6/2, Speed we (rad/s)/1  "Speed estimation"
  Demux6/1 -> Mux18/2
  Psi_r (Noisy)/1 -> V - RI8/2, V - RI7/2
  Demux6/2 -> Gain17/1
  Demux5/1 -> Mux19/2
  Discrete-Time Integrator2/1 -> Psi_r/1, Product6/1, V - RI7/1, V - RI8/1, Demux5/1  "Psi_r"
  Gain16/1 -> V - RI6/2

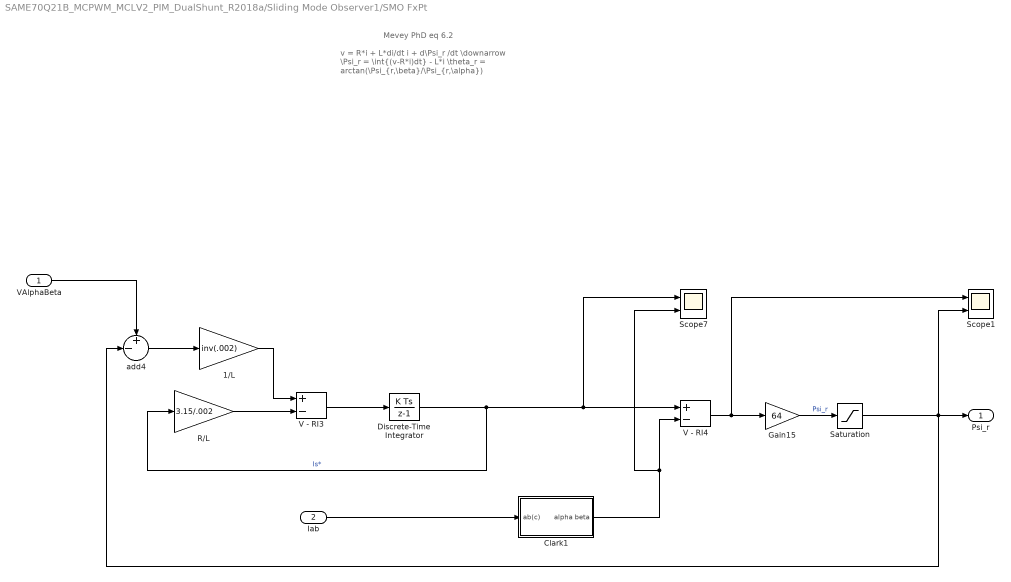
== system SAME70Q21B_MCPWM_MCLV2_PIM_DualShunt_R2018a/Sliding Mode Observer1/SMO FxPt ==
  note: v = R*i + L*di/dt i + d\Psi_r /dt
      | \downarrow
      | \Psi_r = \int{(v-R*i)dt} - L*i
      | \theta_r = arctan(\Psi_{r,\beta}/\Psi_{r,\alpha})
  note: Mevey PhD eq 6.2
  VAlphaBeta : Inport
  Iab : Inport  Port=2
  1/L : Gain  Gain=inv(.002)  OutMin=[-24] * inv(.002) *2  OutMax=[24] * inv(.002) *2  RndMeth=Zero
  Clark1 : Subsystem
  Discrete-Time Integrator : DiscreteIntegrator  SampleTime=-1  OutMin=[-4.4]  OutMax=[4.4]  RndMeth=Zero  ICPrevOutput=DiscIntNeverNeededParam  ICPrevScaledInput=DiscIntNeverNeededParam
  Gain15 : Gain  Gain=64  OutMin=[-24]  OutMax=[24]  RndMeth=Zero
  R/L : Gain  Gain=3.15/.002  OutMin=-4.4*3.15/0.002  OutMax=4.4*3.15/0.002  RndMeth=Zero
  Saturation : Saturate  UpperLimit=32  LowerLimit=-32
  Scope1 : Scope  NumInputPorts=2
  Scope7 : Scope  NumInputPorts=2
  V - RI3 : Sum  Inputs=+-  OutDataTypeStr=Inherit: Same as accumulator  RndMeth=Zero
  V - RI4 : Sum  Inputs=+-  OutMin=-4.4  OutMax=4.4  RndMeth=Zero
  add4 : Sum  Inputs=+-|  OutDataTypeStr=Inherit: Same as accumulator  RndMeth=Zero
  Psi_r : Outport
  wires:
  Saturation/1 -> Psi_r/1, add4/2, Scope1/2
  Gain15/1 -> Saturation/1  "Psi_r"
  Clark1/1(alpha beta) -> Scope7/2, V - RI4/2
  Iab/1 -> Clark1/1(ab(c))
  V - RI4/1 -> Gain15/1, Scope1/1
  Discrete-Time Integrator/1 -> Scope7/1, V - RI4/1, R/L/1  "Is*"
  V - RI3/1 -> Discrete-Time Integrator/1
  VAlphaBeta/1 -> add4/1
  add4/1 -> 1/L/1
  R/L/1 -> V - RI3/2
  1/L/1 -> V - RI3/1

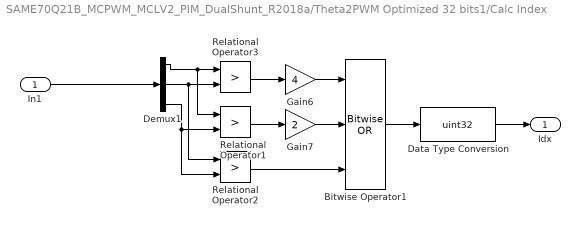
== system SAME70Q21B_MCPWM_MCLV2_PIM_DualShunt_R2018a/Theta2PWM Optimized 32 bits1/Calc Index ==
  In1 : Inport
  Bitwise Operator1 : simulink/Logic and Bit Operations/Bitwise Operator  logicop=OR  UseBitMask=off  NumInputPorts=3  BitMask=bin2dec('11011001')  BitMaskRealWorld=Stored Integer
  Data Type Conversion : DataTypeConversion  OutDataTypeStr=uint32  ConvertRealWorld=Stored Integer (SI)
  Demux1 : Demux  Outputs=3
  Gain6 : Gain  Gain=4  OutDataTypeStr=Inherit: Same as input
  Gain7 : Gain  Gain=2  OutDataTypeStr=Inherit: Same as input
  Relational Operator1 : RelationalOperator  Operator=>  OutDataTypeStr=fixdt(0,32)  RndMeth=Nearest
  Relational Operator2 : RelationalOperator  Operator=>  OutDataTypeStr=fixdt(0,32)  RndMeth=Nearest
  Relational Operator3 : RelationalOperator  Operator=>  OutDataTypeStr=fixdt(0,32)  RndMeth=Nearest
  Idx : Outport
  wires:
  Data Type Conversion/1 -> Idx/1
  In1/1 -> Demux1/1
  Bitwise Operator1/1 -> Data Type Conversion/1
  Demux1/1 -> Relational Operator3/1, Relational Operator1/1
  Relational Operator1/1 -> Gain7/1
  Demux1/3 -> Relational Operator1/2, Relational Operator2/2
  Demux1/2 -> Relational Operator3/2, Relational Operator2/1
  Relational Operator3/1 -> Gain6/1
  Relational Operator2/1 -> Bitwise Operator1/3
  Gain6/1 -> Bitwise Operator1/1
  Gain7/1 -> Bitwise Operator1/2

== system SAME70Q21B_MCPWM_MCLV2_PIM_DualShunt_R2018a/Theta2PWM Optimized 32 bits1/Maximum Duty-Cycle ==
  In1 : Inport
  Constant1 : Constant  Value=PWM0max0  OutDataTypeStr=uint16
  MinMax1 : MinMax  Function=max  OutDataTypeStr=int16  InputSameDT=on
  Sum1 : Sum  Inputs=+-  AccumDataTypeStr=uint16  OutDataTypeStr=Inherit: Same as accumulator  RndMeth=Simplest
  Sum2 : Sum  Inputs=|++  AccumDataTypeStr=uint16  OutDataTypeStr=Inherit: Same as accumulator  RndMeth=Simplest
  Out1 : Outport
  wires:
  Constant1/1 -> Sum1/1
  MinMax1/1 -> Sum1/2
  In1/1 -> Sum2/1, MinMax1/1
  Sum2/1 -> Out1/1
  Sum1/1 -> Sum2/2

== system SAME70Q21B_MCPWM_MCLV2_PIM_DualShunt_R2018a/Theta2PWM Optimized 32 bits1/Minimum Duty-Cycle ==
  In1 : Inport
  Bias : Bias  Bias=-round( (2e-6/5e-5) *PWM0max0 )
  MinMax1 : MinMax  OutDataTypeStr=int16  InputSameDT=on
  Sum2 : Sum  Inputs=|+-  AccumDataTypeStr=uint16  OutDataTypeStr=Inherit: Same as accumulator  RndMeth=Simplest
  Out1 : Outport
  wires:
  In1/1 -> MinMax1/1, Sum2/1
  Sum2/1 -> Out1/1
  MinMax1/1 -> Bias/1
  Bias/1 -> Sum2/2

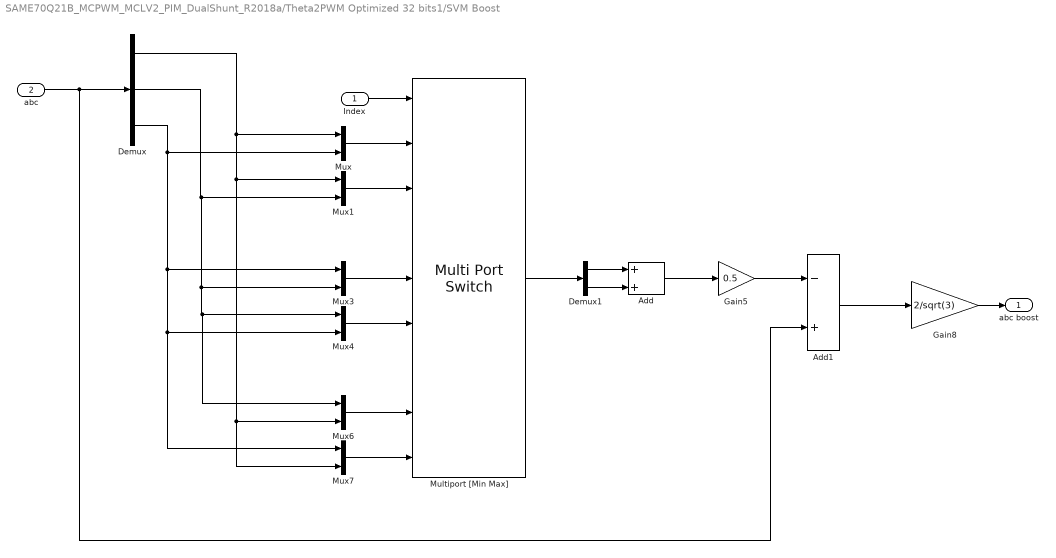
== system SAME70Q21B_MCPWM_MCLV2_PIM_DualShunt_R2018a/Theta2PWM Optimized 32 bits1/SVM Boost ==
  Index : Inport
  abc : Inport  Port=2
  Add : Sum  OutDataTypeStr=Inherit: Same as accumulator  RndMeth=Zero
  Add1 : Sum  Inputs=-+  RndMeth=Zero  OutDataTypeStr=Inherit: Same as first input
  Demux : Demux  Outputs=3
  Demux1 : Demux  Outputs=2
  Gain5 : Gain  Gain=0.5  RndMeth=Zero  OutDataTypeStr=Inherit: Same as input
  Gain8 : Gain  Gain=2/sqrt(3)  RndMeth=Zero  ParamDataTypeStr=Inherit: Same as input
  Multiport [Min Max] : MultiPortSwitch  DataPortOrder=Zero-based contiguous  Inputs=8  DiagnosticForDefault=None  zeroidx=on
  Mux{,1,3..4,6..7} (6 alike) : Mux  Inputs=2
  abc boost : Outport
  wires:
  Add/1 -> Gain5/1
  Gain5/1 -> Add1/1
  Add1/1 -> Gain8/1
  abc/1 -> Add1/2, Demux/1
  Gain8/1 -> abc boost/1
  Index/1 -> Multiport [Min Max]/1
  Mux/1 -> Multiport [Min Max]/2
  Mux1/1 -> Multiport [Min Max]/3
  Mux3/1 -> Multiport [Min Max]/5
  Mux4/1 -> Multiport [Min Max]/6
  Mux6/1 -> Multiport [Min Max]/8
  Mux7/1 -> Multiport [Min Max]/9
  Demux/1 -> Mux7/2, Mux6/2, Mux1/1, Mux/1
  Demux/3 -> Mux/2, Mux3/1, Mux4/2, Mux7/1
  Demux/2 -> Mux6/1, Mux4/1, Mux3/2, Mux1/2
  Multiport [Min Max]/1 -> Demux1/1
  Demux1/1 -> Add/1
  Demux1/2 -> Add/2

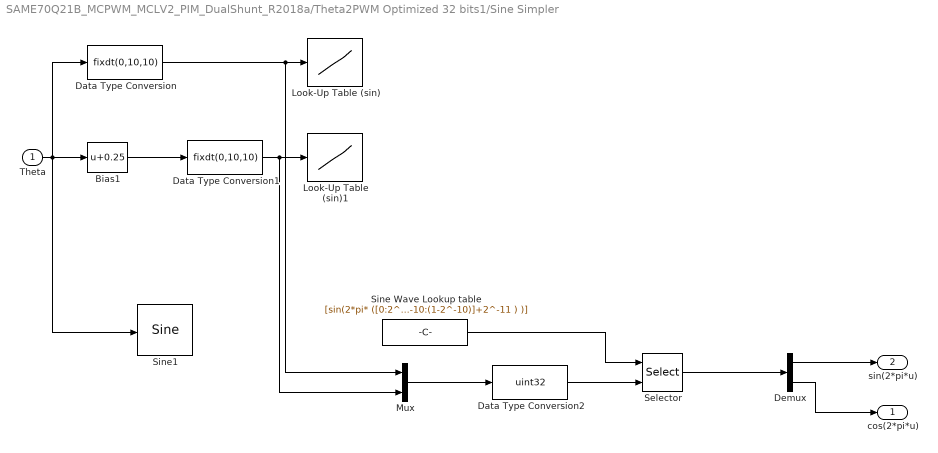
== system SAME70Q21B_MCPWM_MCLV2_PIM_DualShunt_R2018a/Theta2PWM Optimized 32 bits1/Sine Simpler ==
  Theta : Inport
  Bias1 : Bias  Bias=0.25
  Data Type Conversion : DataTypeConversion  OutDataTypeStr=fixdt(0,10,10)
  Data Type Conversion1 : DataTypeConversion  OutDataTypeStr=fixdt(0,10,10)
  Data Type Conversion2 : DataTypeConversion  OutDataTypeStr=uint32  ConvertRealWorld=Stored Integer (SI)
  Demux : Demux  Outputs=2
  Look-Up Table (sin) : Lookup_n-D  NumberOfTableDimensions=1  BreakpointsSpecification=Even spacing  BreakpointsForDimension1=XData  BreakpointsForDimension1FirstPoint=0  BreakpointsForDimension1Spacing=2^-10  IndexSearchMethod=Evenly spaced points  Table=sin(2*pi* ([0:2^-10:(1-2^-10)]+2^-11 ) )  InterpMethod=Flat  ExtrapMethod=Clip  RemoveProtectionInput=on  InternalRulePriority=Speed  OutDataTypeStr=fixdt(1, 32, 30)  RndMeth=Zero  LockScale=on
  Look-Up Table (sin)1 : Lookup_n-D  NumberOfTableDimensions=1  BreakpointsSpecification=Even spacing  BreakpointsForDimension1=XData  BreakpointsForDimension1FirstPoint=0  BreakpointsForDimension1Spacing=2^-10  IndexSearchMethod=Evenly spaced points  Table=sin(2*pi* ([0:2^-10:(1-2^-10)]+2^-11 ) )  InterpMethod=Flat  ExtrapMethod=Clip  RemoveProtectionInput=on  InternalRulePriority=Speed  OutDataTypeStr=fixdt(1, 32, 30)  RndMeth=Zero  LockScale=on
  Mux : Mux  Inputs=2
  Selector : Selector  IndexMode=Zero-based  InputPortWidth=1024  IndexOptions=Index vector (port)  Indices=[1 3]  OutputSizes=1
  Sine Wave Lookup table : Constant  Value=[sin(2*pi* ([0:2^-10:(1-2^-10)]+2^-11 ) )]  OutDataTypeStr=double
  Sine1 : simulink/Lookup Tables/Sine  Formula=sin(2*pi*u) and cos(2*pi*u)  NumDataPoints=(2^5)+1  OutputWordLength=16  InternalRulePriority=Speed
      settings: SourceProductName=Simulink
  cos(2*pi*u) : Outport
  sin(2*pi*u) : Outport  Port=2
  wires:
  Demux/2 -> cos(2*pi*u)/1
  Demux/1 -> sin(2*pi*u)/1
  Selector/1 -> Demux/1
  Data Type Conversion2/1 -> Selector/2
  Mux/1 -> Data Type Conversion2/1
  Sine Wave Lookup table/1 -> Selector/1
  Data Type Conversion1/1 -> Look-Up Table (sin)1/1, Mux/2
  Data Type Conversion/1 -> Look-Up Table (sin)/1, Mux/1
  Theta/1 -> Sine1/1, Data Type Conversion/1, Bias1/1
  Bias1/1 -> Data Type Conversion1/1

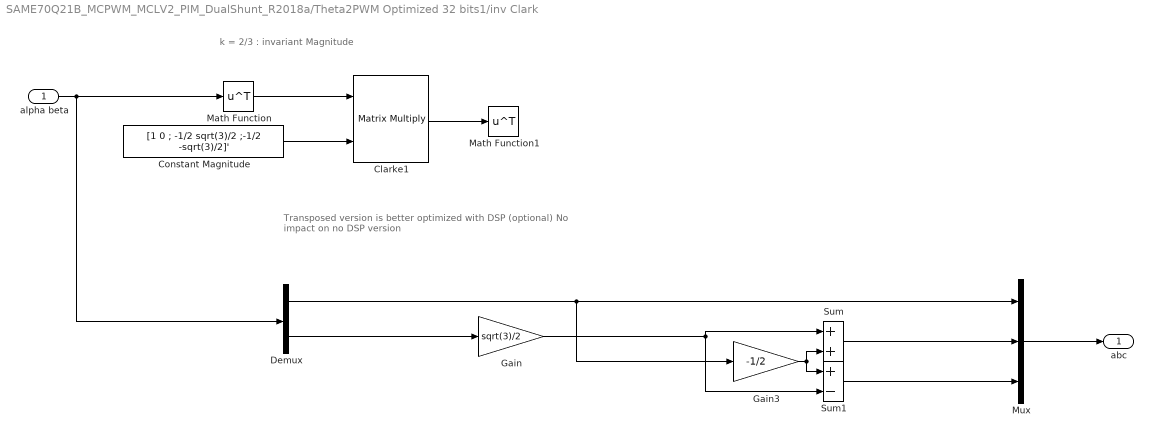
== system SAME70Q21B_MCPWM_MCLV2_PIM_DualShunt_R2018a/Theta2PWM Optimized 32 bits1/inv Clark ==
  note: Transposed version is better optimized with DSP (optional)
      | No impact on no DSP version
  note: k = 2/3 : invariant Magnitude
  alpha beta : Inport
  Clarke1 : Product  Multiplication=Matrix(*)  RndMeth=Simplest  OutDataTypeStr=Inherit: Same as first input
  Constant Magnitude : Constant  Value=[1 0 ; -1/2 sqrt(3)/2 ;-1/2 -sqrt(3)/2]'  OutDataTypeStr=Inherit: Inherit via back propagation  SampleTime=-1
  Demux : Demux  Outputs=2
  Gain : Gain  Gain=sqrt(3)/2  OutDataTypeStr=Inherit: Inherit via back propagation  RndMeth=Zero
  Gain3 : Gain  Gain=-1/2  OutDataTypeStr=Inherit: Inherit via back propagation  RndMeth=Zero
  Math Function : Math  Operator=transpose  SaturateOnIntegerOverflow=on
  Math Function1 : Math  Operator=transpose  SaturateOnIntegerOverflow=on
  Mux : Mux  Inputs=3
  Sum : Sum  RndMeth=Zero  OutDataTypeStr=Inherit: Same as first input
  Sum1 : Sum  Inputs=+-  RndMeth=Zero  SaturateOnIntegerOverflow=on  OutDataTypeStr=Inherit: Same as first input
  abc : Outport
  wires:
  Demux/1 -> Gain3/1, Mux/1
  Demux/2 -> Gain/1
  Constant Magnitude/1 -> Clarke1/2
  alpha beta/1 -> Math Function/1, Demux/1
  Gain/1 -> Sum1/2, Sum/1
  Sum/1 -> Mux/2
  Sum1/1 -> Mux/3
  Gain3/1 -> Sum1/1, Sum/2
  Clarke1/1 -> Math Function1/1
  Math Function/1 -> Clarke1/1
  Mux/1 -> abc/1

== system SAME70Q21B_MCPWM_MCLV2_PIM_DualShunt_R2018a/Sliding Mode Observer1/Atan x2/abs ==
  In3 : Inport
  Compare To Zero : simulink/Logic and Bit Operations/Compare To Zero  relop=>=  OutDataTypeStr=boolean
  Gain : Gain  Gain=-1  OutDataTypeStr=Inherit: Same as input
  Switch2 : Switch  Criteria=u2 ~= 0
  abs : Outport
  sign : Outport  Port=2
  wires:
  Compare To Zero/1 -> Switch2/2, sign/1
  In3/1 -> Compare To Zero/1, Switch2/1, Gain/1
  Gain/1 -> Switch2/3
  Switch2/1 -> abs/1

== system SAME70Q21B_MCPWM_MCLV2_PIM_DualShunt_R2018a/Sliding Mode Observer1/Atan x2/abs1 ==
  In3 : Inport
  Compare To Zero : simulink/Logic and Bit Operations/Compare To Zero  relop=>=  OutDataTypeStr=boolean
  Gain : Gain  Gain=-1  OutDataTypeStr=Inherit: Same as input
  Switch2 : Switch  Criteria=u2 ~= 0
  abs : Outport
  sign : Outport  Port=2
  wires:
  Switch2/1 -> abs/1
  Gain/1 -> Switch2/3
  In3/1 -> Gain/1, Switch2/1, Compare To Zero/1
  Compare To Zero/1 -> sign/1, Switch2/2

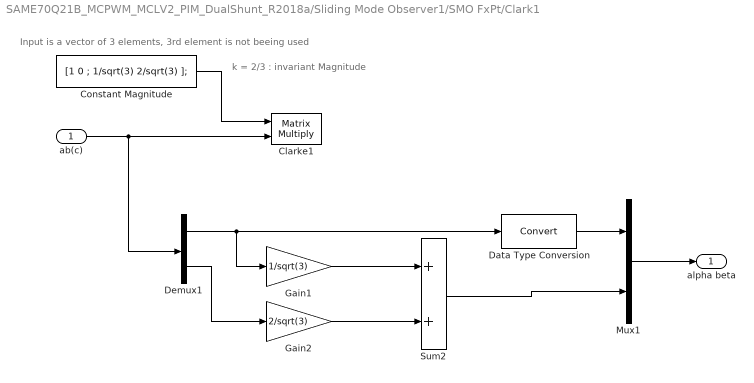
== system SAME70Q21B_MCPWM_MCLV2_PIM_DualShunt_R2018a/Sliding Mode Observer1/SMO FxPt/Clark1 ==
  note: k = 2/3 : invariant Magnitude
  note: Input is a vector of 3 elements, 3rd element is not beeing used
  ab(c) : Inport
  Clarke1 : Product  Multiplication=Matrix(*)  OutMin=[-4.4]  OutMax=[4.4]  OutDataTypeStr=fixdt(1,16)  SaturateOnIntegerOverflow=on  RndMeth=Zero
  Constant Magnitude : Constant  Value=[1 0 ; 1/sqrt(3) 2/sqrt(3) ];  OutDataTypeStr=fixdt(1,16)
  Data Type Conversion : DataTypeConversion  RndMeth=Zero
  Demux1 : Demux  Outputs=2
  Gain1 : Gain  Gain=1/sqrt(3)  OutMin=[-4.4]  OutMax=[4.4]  OutDataTypeStr=double  RndMeth=Zero
  Gain2 : Gain  Gain=2/sqrt(3)  OutMin=[-4.4]  OutMax=[4.4]  OutDataTypeStr=double  RndMeth=Zero
  Mux1 : Mux  Inputs=2
  Sum2 : Sum  RndMeth=Zero  OutDataTypeStr=Inherit: Same as first input
  alpha beta : Outport
  wires:
  Data Type Conversion/1 -> Mux1/1
  Mux1/1 -> alpha beta/1
  Sum2/1 -> Mux1/2
  Gain2/1 -> Sum2/2
  Gain1/1 -> Sum2/1
  Demux1/2 -> Gain2/1
  Demux1/1 -> Data Type Conversion/1, Gain1/1
  Constant Magnitude/1 -> Clarke1/1
  ab(c)/1 -> Clarke1/2, Demux1/1
